simulink model "LAB2_Delta"  (R2020a)
settings: Solver=VariableStepAuto  StartTime=0.0  StopTime=10.0  RelTol=1e-3
libraries: dspquant2 x2, dsparch4 x1, dspsrcs4 x1
settings Model: Creator=Sameer  LastModifiedBy=Sameer

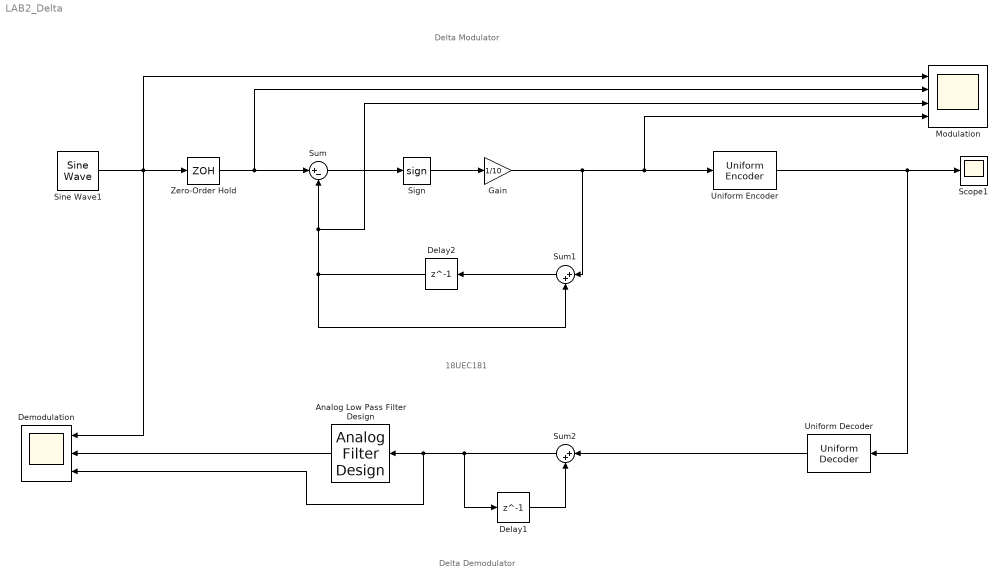
== system LAB2_Delta ==
  note: 18UEC181
  note: Delta Demodulator
  note: Delta Modulator
  Analog Low Pass Filter Design : dsparch4/Analog Filter Design  method=Butterworth  filttype=Lowpass  N=8  Wlo=2*pi  Whi=80  Rp=2  Rs=40
  Delay1 : Delay  DelayLength=1
  Delay2 : Delay  DelayLength=1
  Demodulation : Scope  NumInputPorts=3
  Gain : Gain  Gain=1/10
  Modulation : Scope  NumInputPorts=4
  Scope1 : Scope
  Sign : Signum
  Sine Wave1 : dspsrcs4/Sine Wave  Amplitude=5  Frequency=1  Phase=0  SampleMode=Discrete  OutComplex=Real  CompMethod=Trigonometric fcn  TableSize=Speed  SampleTime=1/1000  SamplesPerFrame=1  ResetState=Restart at time zero  OutputFrames=off  dataType=double  wordLen=16  udDataType=sfix(16)  fracBitsMode=Best precision  numFracBits=15  OutDataTypeStr=double  LastOutDataTypeStr=double
  Sum : Sum  Inputs=|+-
  Sum1 : Sum  Inputs=|++
  Sum2 : Sum  Inputs=|++
  Uniform Decoder : dspquant2/Uniform Decoder  peak=1  bits=8  overflowMode=Saturate  otype=Double
      settings: SourceProductBaseCode=DS
  Uniform Encoder : dspquant2/Uniform Encoder  peak=1  bits=8  otype=Unsigned integer
  Zero-Order Hold : ZeroOrderHold  SampleTime=1/20
  wires:
  Sine Wave1/1 -> Demodulation/1, Modulation/1, Zero-Order Hold/1
  Zero-Order Hold/1 -> Modulation/2, Sum/1
  Uniform Encoder/1 -> Uniform Decoder/1, Scope1/1
  Analog Low Pass Filter Design/1 -> Demodulation/2
  Uniform Decoder/1 -> Sum2/1
  Sum2/1 -> Demodulation/3, Analog Low Pass Filter Design/1, Delay1/1
  Delay1/1 -> Sum2/2
  Sign/1 -> Gain/1
  Sum/1 -> Sign/1
  Gain/1 -> Sum1/1, Uniform Encoder/1, Modulation/4
  Sum1/1 -> Delay2/1
  Delay2/1 -> Modulation/3, Sum/2, Sum1/2
